simulink model "oel2"  (R2020a)
settings: Solver=VariableStepAuto  StartTime=0.0  StopTime=5  RelTol=1e-3
libraries: powerlib x27
settings Model: Creator=Dell  LastModifiedBy=Dell

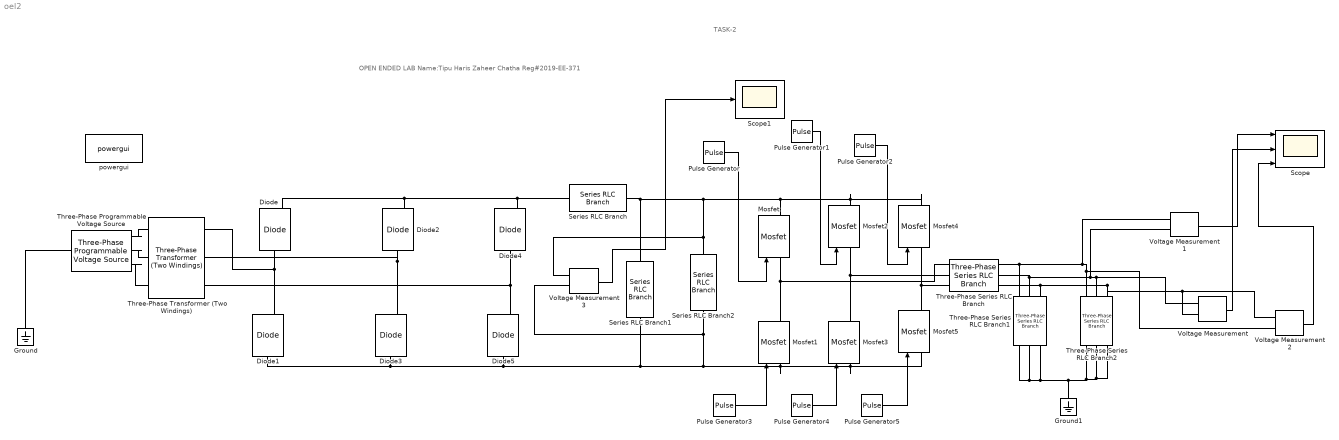
== system oel2 ==
  note: OPEN ENDED LAB
      | Name:Tipu Haris Zaheer Chatha
      | Reg#2019-EE-371
  note: TASK-2
  Diode{,1..5} (6 alike) : powerlib/Power Electronics/Diode  Ron=0.001  Lon=0  Vf=0.8  IC=0  UseSnubber=0  Rs=500  Cs=250e-9  Measurements=on
  Ground : powerlib/Elements/Ground  LConnTagsString=a
  Ground1 : powerlib/Elements/Ground  LConnTagsString=a
  Mosfet{,1..5} (6 alike) : powerlib/Power Electronics/Mosfet  Ron=0.1  Lon=0  Rd=0.01  Vfd=0  IC=0  Rs=1e5  Cs=inf  Measurements=on
  Pulse Generator : DiscretePulseGenerator  PulseType=Time based  Period=1/20  PulseWidth=50  PhaseDelay=0/(130*360)
  Pulse Generator1 : DiscretePulseGenerator  PulseType=Time based  Period=1/20  PulseWidth=50  PhaseDelay=120/(20*360)
  Pulse Generator2 : DiscretePulseGenerator  PulseType=Time based  Period=1/20  PulseWidth=50  PhaseDelay=240/(20*360)
  Pulse Generator3 : DiscretePulseGenerator  PulseType=Time based  Period=1/20  PulseWidth=50  PhaseDelay=180/(20*360)
  Pulse Generator4 : DiscretePulseGenerator  PulseType=Time based  Period=1/20  PulseWidth=50  PhaseDelay=300/(20*360)
  Pulse Generator5 : DiscretePulseGenerator  PulseType=Time based  Period=1/20  PulseWidth=50  PhaseDelay=60/(50*360)
  Scope : Scope  NumInputPorts=3
  Scope1 : Scope
  Series RLC Branch : powerlib/Elements/Series RLC Branch  LConnTagsString=__new0  RConnTagsString=__new0  BranchType=L  Resistance=1  Inductance=1e-3  SetiL0=off  InitialCurrent=0  Capacitance=1e-6  Setx0=off  InitialVoltage=0  Measurements=None
  Series RLC Branch1 : powerlib/Elements/Series RLC Branch  LConnTagsString=__new0  RConnTagsString=__new0  BranchType=C  Resistance=1  Inductance=1e-3  SetiL0=off  InitialCurrent=0  Capacitance=0.01013  Setx0=off  InitialVoltage=0  Measurements=None
  Series RLC Branch2 : powerlib/Elements/Series RLC Branch  LConnTagsString=__new0  RConnTagsString=__new0  BranchType=R  Resistance=50  Inductance=1e-3  SetiL0=off  InitialCurrent=0  Capacitance=1e-6  Setx0=off  InitialVoltage=0  Measurements=None
  Three-Phase Programmable Voltage Source : powerlib/Electrical Sources/Three-Phase Programmable Voltage Source  PositiveSequence="[230  0 50]"  VariationEntity=None  VariationType=Table of time-amplitude pairs  VariationTypeAlt=Step  VariationStep=0.5  VariationRate=10  VariationMagnitude=0.3  VariationFrequency=2  VariationTiming=[1 2]  VariationPhaseA=off  Amplitudes=[1 0.8 1.2 1.0]  TimeValues=[0 0.1 0.15 0.2]  HarmonicGeneration=off  HarmonicA=[3 0.2 -25 0]  HarmonicB=[2 0.15 35 2]  Timing="[0.05  3]"  BusType=swing  Pref=0  Qref=0  Qmin=-inf  Qmax=inf
  Three-Phase Series RLC Branch : powerlib/Elements/Three-Phase Series RLC Branch  LConnTagsString=A|B|C  RConnTagsString=A|B|C  BranchType=L  Resistance=1  Inductance=1e-3  Capacitance=1e-6  Measurements=None
  Three-Phase Series RLC Branch1 : powerlib/Elements/Three-Phase Series RLC Branch  LConnTagsString=A|B|C  RConnTagsString=A|B|C  BranchType=C  Resistance=1  Inductance=1e-3  Capacitance=0.06332  Measurements=None
  Three-Phase Series RLC Branch2 : powerlib/Elements/Three-Phase Series RLC Branch  LConnTagsString=A|B|C  RConnTagsString=A|B|C  BranchType=R  Resistance=25  Inductance=1e-3  Capacitance=1e-6  Measurements=None
  Three-Phase Transformer (Two Windings) : powerlib/Elements/Three-Phase Transformer (Two Windings)  Winding1Connection=Yg  Winding2Connection=Yg  CoreType=Three single-phase transformers  SetSaturation=off  Hysteresis=off  DataFile='hysteresis'  SetInitialFlux=off  Measurements=None  UNITS=SI  NominalPower=[ 250e6 , 50 ]  Winding1=[230 0 0]  Winding2=[610 0 0]  Rm=1.0805e+06  Lm=2866  L0=0.5  Saturation=[0 0;0.66653 1910.3;277.72 2419.7]  InitialFluxes=[ 0.8 , -0.8 , 0.7 ]  BreakLoop=off  DiscreteSolver=Trapezoidal iterative  DataType=on  TransfoNumber=1
  Voltage Measurement{,1..3} (4 alike) : powerlib/Measurements/Voltage Measurement  PhasorSimulation=off  OutputType=Complex  PSBequivalent=0
  powergui : powerlib/powergui  Priority=1  SimulationMode=Continuous  SampleTime=50e-6  frequency=60  Iterations=50  frequencyindice=50  Pbase=100e6  ErrMax=1e-4  UnitsV=kV  UnitsW=MW  buscounter=0  FunctionMessages=off  echomessages=off  EnableUseOfTLC=off  CurrentSourceSwitches=off  DisableSnubberDevices=off  DisableRonSwitches=off  DisableVfSwitches=off  DisplayEquations=off  AutomaticDiscreteSolvers=off  SolverType=Tustin/Backward Euler (TBE)  Interpol=off  ExternalGateDelay=off  methode=off  Ts=100  x0status=blocks  SPID=on  SwTol=0  HookPort=off  NonlinearTolerance=1e-4  nMaxIteration=100  ContinueOnMaxIteration=off  RestoreLinks=warning  ResistiveCurrentMeasurement=off  Frange=[0:2:500]  Ylog=off  Xlog=on  ShowGrid=off  save=off  variable=ZData  structure=0  ZoomFFT=off  StartTime=0.0  cycles=1  DisplayStyle=1  fundamental=60  FreqAxis=off  MaxFrequency=1000  frequencyindicesteady=1  RmsSteady=1  display=off
  wires:
  Voltage Measurement3/1 -> Scope1/1
  Voltage Measurement2/1 -> Scope/3
  Voltage Measurement1/1 -> Scope/1
  Voltage Measurement/1 -> Scope/2
  Pulse Generator4/1 -> Mosfet3/1
  Pulse Generator3/1 -> Mosfet1/1
  Pulse Generator2/1 -> Mosfet4/1
  Pulse Generator/1 -> Mosfet/1
  Pulse Generator1/1 -> Mosfet2/1
  Pulse Generator5/1 -> Mosfet5/1
  connections:
  Three-Phase Series RLC Branch2/LConn2 -- Voltage Measurement/LConn1 -- Voltage Measurement1/LConn2 -- Three-Phase Series RLC Branch1/LConn2 -- Three-Phase Series RLC Branch/RConn2
  Diode3/RConn1 -- Three-Phase Transformer (Two Windings)/RConn2 -- Diode2/LConn1
  Three-Phase Series RLC Branch2/LConn3 -- Voltage Measurement/LConn2 -- Voltage Measurement2/LConn1 -- Three-Phase Series RLC Branch1/LConn3 -- Three-Phase Series RLC Branch/RConn3
  Mosfet/RConn1 -- Voltage Measurement3/LConn1 -- Series RLC Branch2/RConn1 -- Series RLC Branch1/LConn1 -- Series RLC Branch/RConn1 -- Mosfet4/RConn1 -- Mosfet2/RConn1
  Three-Phase Series RLC Branch2/RConn1 -- Three-Phase Series RLC Branch2/RConn3 -- Three-Phase Series RLC Branch2/RConn2 -- Three-Phase Series RLC Branch1/RConn3 -- Three-Phase Series RLC Branch1/RConn2 -- Three-Phase Series RLC Branch1/RConn1 -- Ground1/LConn1
  Mosfet1/LConn1 -- Mosfet5/LConn1 -- Mosfet3/LConn1 -- Voltage Measurement3/LConn2 -- Series RLC Branch2/LConn1 -- Series RLC Branch1/RConn1 -- Diode1/LConn1 -- Diode3/LConn1 -- Diode5/LConn1
  Mosfet2/LConn1 -- Mosfet3/RConn1 -- Three-Phase Series RLC Branch/LConn2
  Three-Phase Series RLC Branch/RConn1 -- Three-Phase Series RLC Branch1/LConn1 -- Voltage Measurement1/LConn1 -- Voltage Measurement2/LConn2 -- Three-Phase Series RLC Branch2/LConn1
  Diode5/RConn1 -- Three-Phase Transformer (Two Windings)/RConn3 -- Diode4/LConn1
  Diode4/RConn1 -- Diode/RConn1 -- Diode2/RConn1 -- Series RLC Branch/LConn1
  Diode1/RConn1 -- Three-Phase Transformer (Two Windings)/RConn1 -- Diode/LConn1
  Mosfet4/LConn1 -- Mosfet5/RConn1 -- Three-Phase Series RLC Branch/LConn3
  Mosfet/LConn1 -- Mosfet1/RConn1 -- Three-Phase Series RLC Branch/LConn1
  Three-Phase Programmable Voltage Source/RConn1 -- Three-Phase Transformer (Two Windings)/LConn1
  Three-Phase Programmable Voltage Source/RConn2 -- Three-Phase Transformer (Two Windings)/LConn2
  Three-Phase Programmable Voltage Source/RConn3 -- Three-Phase Transformer (Two Windings)/LConn3
  Ground/LConn1 -- Three-Phase Programmable Voltage Source/LConn1
